simulink model "partB"  (R2022b)
settings: Solver=VariableStepAuto  StartTime=0.0  StopTime=10.0  RelTol=1e-3
undefined symbols (not defined in the file or in its folder): A_c, k_a
libraries: simulink x1
settings Model: Creator=kareem  LastModifiedBy=kareem

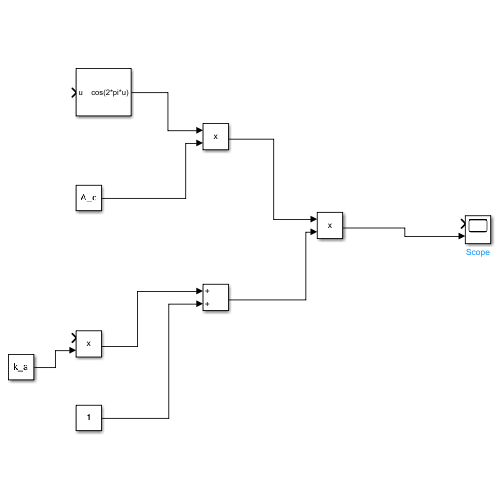
[thumbnail: Simulink's stored preview of the top-level diagram]
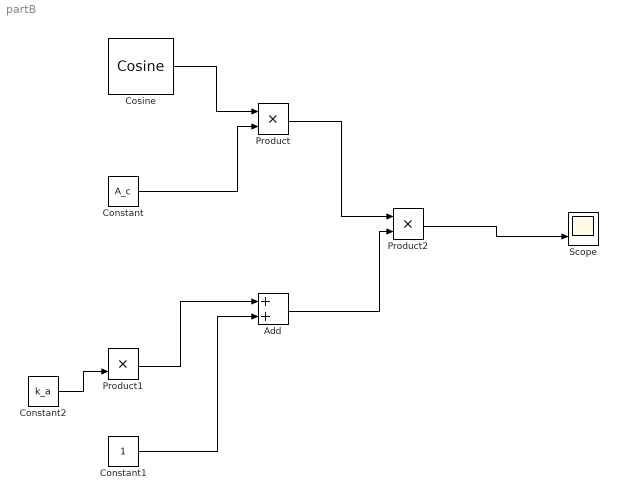
== system partB ==
  Add : Sum
  Constant : Constant  Value=A_c
  Constant1 : Constant
  Constant2 : Constant  Value=k_a
  Cosine : simulink/Lookup Tables/Cosine  Formula=cos(2*pi*u)  NumDataPoints=(2^5)+1  OutputWordLength=16  InternalRulePriority=Speed
  Product : Product
  Product1 : Product
  Product2 : Product
  Scope : Scope  NumInputPorts=2
  wires:
  Cosine/1 -> Product/1
  Constant/1 -> Product/2
  Constant1/1 -> Add/2
  Constant2/1 -> Product1/2
  Product1/1 -> Add/1
  Product/1 -> Product2/1
  Add/1 -> Product2/2
  Product2/1 -> Scope/2
